simulink model "provaikine"  (R2016a)
settings: Solver=VariableStepAuto  StartTime=0.0  StopTime=10.0  RelTol=1e-3
libraries: WBToolboxLibrary x4
settings Model: Creator=sdafarra  LastModifiedBy=sdafarra

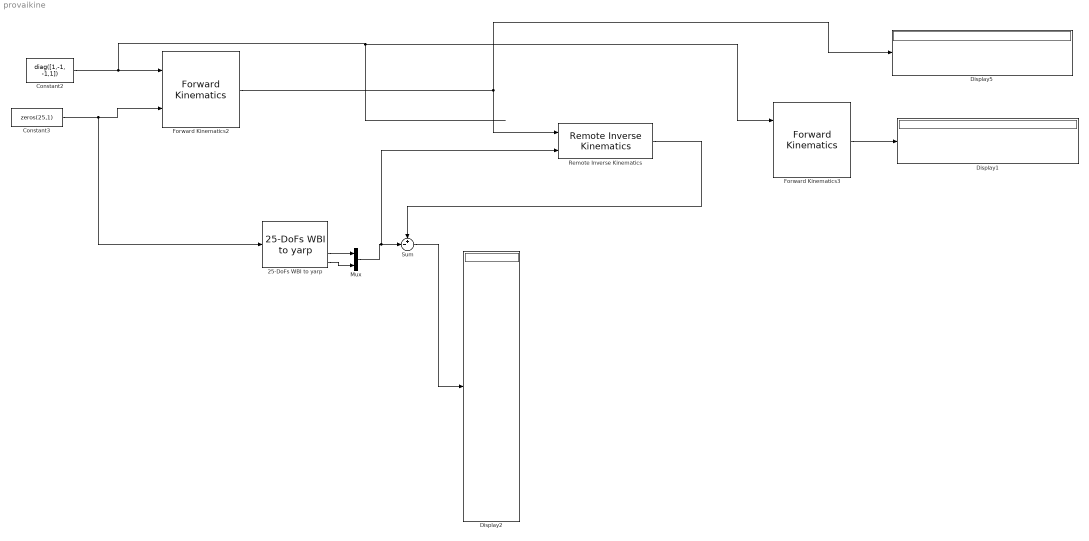
== system provaikine ==
  25-DoFs WBI to yarp : WBToolboxLibrary/Utilities/25-DoFs WBI to yarp
  Constant2 : Constant  Value=diag([1,-1, -1,1])
  Constant3 : Constant  Value=zeros(25,1)
  Display1 : Display
  Display2 : Display
  Display5 : Display
  Forward Kinematics2 : WBToolboxLibrary/wholeBodyModel/Kinematics/Forward Kinematics  frameName='r_sole'  robotName=WBT_robotName  localName=WBT_modelName  wbiFile=WBT_wbiFilename  wbiList=WBT_wbiList
  Forward Kinematics3 : WBToolboxLibrary/wholeBodyModel/Kinematics/Forward Kinematics  frameName='r_sole'  robotName=WBT_robotName  localName=WBT_modelName  wbiFile=WBT_wbiFilename  wbiList=WBT_wbiList
  Mux : Mux  Inputs=2
  Remote Inverse Kinematics : WBToolboxLibrary/wholeBodyModel/Kinematics/Remote Inverse Kinematics  solverName='/cartesianSolver'  dofs=12  optOption=Full Constraint (Position and Orientation)
  Sum : Sum  Inputs=+-|
  wires:
  Constant3/1 -> 25-DoFs WBI to yarp/1, Forward Kinematics2/2
  Sum/1 -> Display2/1
  Forward Kinematics2/1 -> Remote Inverse Kinematics/1, Display5/1
  Remote Inverse Kinematics/1 -> Sum/1
  Constant2/1 -> Forward Kinematics3/1, Forward Kinematics2/1
  Forward Kinematics3/1 -> Display1/1
  25-DoFs WBI to yarp/4 -> Mux/1
  25-DoFs WBI to yarp/5 -> Mux/2
  Mux/1 -> Remote Inverse Kinematics/2, Sum/2
